simulink model "HW5_Q1sim"  (R2023a)
settings: Solver=VariableStepAuto  StartTime=0.0  StopTime=10.0  RelTol=1e-3
values from neighbouring files (symbols this model uses):
  Bm = 1*10^-5    (= 1e-05)    [HW5_Group3_1_1.m]    (also in HW5_Group3_1_2.m = 1e-08)
  JL = Jb+m*l^2    (= 0.0001002)    [HW5_Group3_1_1.m]
  Jm = 3*10^-5    (= 3e-05)    [HW5_Group3_1_1.m]    (also in HW5_Group3_1_2.m = 2.5e-05)
  Km = 3*10^-2    (= 0.03)    [HW5_Group3_1_1.m]    (also in HW5_Group3_1_2.m = 0.066)
  r = 10    [HW5_Group3_1_1.m]    (also in HW5_Group3_1_2.m = 6.25)
  Rm = 6    [HW5_Group3_1_1.m]    (also in HW5_Group3_1_2.m = 4.8)
settings Model: Creator=USER  LastModifiedBy=USER

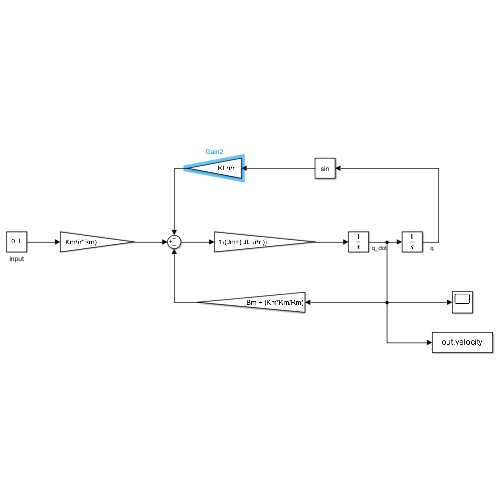
[thumbnail: Simulink's stored preview of the top-level diagram]
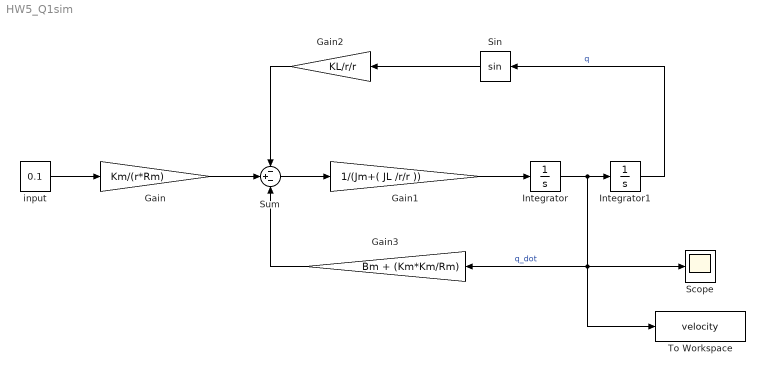
== system HW5_Q1sim ==
  Gain : Gain  Gain=Km/(r*Rm)
  Gain1 : Gain  Gain=1/(Jm+( JL /r/r ))
  Gain2 : Gain  Gain=KL/r/r
  Gain3 : Gain  Gain=Bm + (Km*Km/Rm)
  Integrator : Integrator
  Integrator1 : Integrator
  Scope : Scope
  Sin : Trigonometry
  Sum : Sum  Inputs=-+-
  To Workspace : ToWorkspace  VariableName=velocity  SaveFormat=Timeseries  SampleTime=-1
  input : Constant  Value=0.1
  wires:
  Gain/1 -> Sum/2
  input/1 -> Gain/1
  Integrator/1 -> To Workspace/1, Gain3/1, Scope/1, Integrator1/1  "q_dot"
  Gain1/1 -> Integrator/1
  Sum/1 -> Gain1/1
  Integrator1/1 -> Sin/1  "q"
  Sin/1 -> Gain2/1
  Gain2/1 -> Sum/1
  Gain3/1 -> Sum/3
